simulink model "LB01B01"  (R2022b)
settings: Solver=ode45  StartTime=0.0  StopTime=20.0  MaxStep=0.01  RelTol=1e-3
settings Model: Creator=Andrey  LastModifiedBy=Andrey

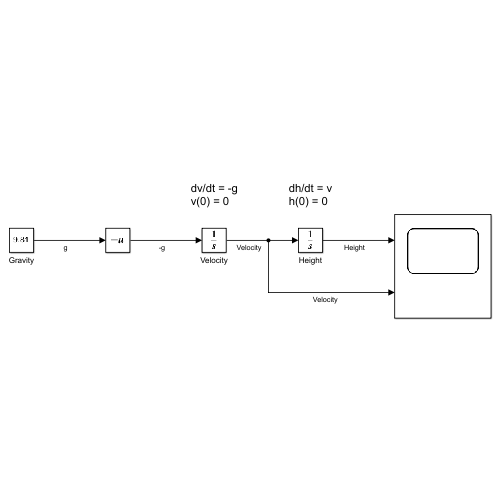
[thumbnail: Simulink's stored preview of the top-level diagram]
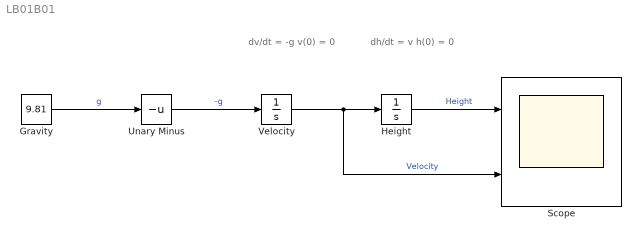
== system LB01B01 ==
  note: dh/dt = v
      | h(0) = 0
  note: dv/dt = -g
      | v(0) = 0
  Gravity : Constant  Value=9.81
  Height : Integrator
  Scope : Scope  NumInputPorts=2
  Unary Minus : UnaryMinus
  Velocity : Integrator
  wires:
  Gravity/1 -> Unary Minus/1  "g"
  Unary Minus/1 -> Velocity/1  "-g"
  Velocity/1 -> Scope/2, Height/1  "Velocity"
  Height/1 -> Scope/1  "Height"
